simulink model "simulation_model"  (R2019b)
settings: Solver=VariableStepAuto  StartTime=0.0  StopTime=3  RelTol=1e-3
values from neighbouring files (symbols this model uses):
  g = 9.80665    [main.m]
  h = 0.5    [main.m]
  kv = 0.1    [main.m]
  m = 30 * 10^-3    (= 0.03)    [main.m]
  v0_x = v0 * cos(theta)    [main.m]
  v0_y = v0 * sin(theta)    [main.m]
libraries: simulink x1
settings Model: Creator=super  LastModifiedBy=super

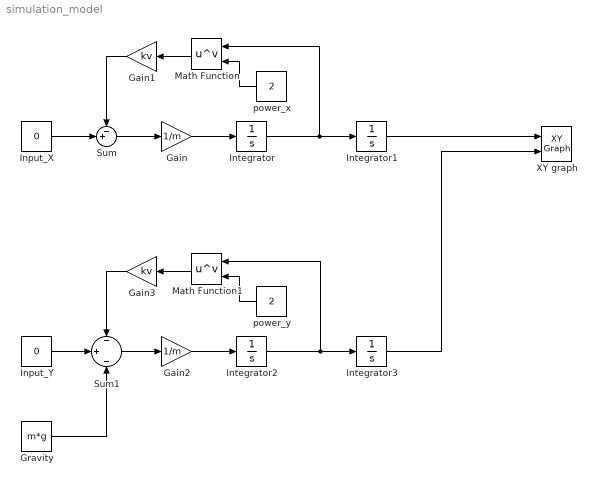
== system simulation_model ==
  Gain : Gain  Gain=1/m
  Gain1 : Gain  Gain=kv
  Gain2 : Gain  Gain=1/m
  Gain3 : Gain  Gain=kv
  Gravity : Constant  Value=m*g
  Input_X : Constant  Value=0
  Input_Y : Constant  Value=0
  Integrator : Integrator  InitialCondition=v0_x  LimitOutput=on  LowerSaturationLimit=0
  Integrator1 : Integrator
  Integrator2 : Integrator  InitialCondition=v0_y  LimitOutput=on  UpperSaturationLimit=10^3  LowerSaturationLimit=-10^3
  Integrator3 : Integrator  InitialCondition=h  LimitOutput=on  LowerSaturationLimit=0
  Math Function : Math  Operator=pow  SignedPower=off  SaturateOnIntegerOverflow=on
  Math Function1 : Math  Operator=pow  SignedPower=off  SaturateOnIntegerOverflow=on
  Sum : Sum  Inputs=-+|
  Sum1 : Sum  Inputs=-|+|-
  XY graph : simulink/Sinks/XY Graph  xmin=-1  xmax=5  ymin=0  ymax=1  st=-1
  power_x : Constant  Value=2
  power_y : Constant  Value=2
  wires:
  Sum/1 -> Gain/1
  Input_X/1 -> Sum/2
  Gain/1 -> Integrator/1
  Integrator/1 -> Math Function/1, Integrator1/1
  power_x/1 -> Math Function/2
  Math Function/1 -> Gain1/1
  Gain1/1 -> Sum/1
  Math Function1/1 -> Gain3/1
  power_y/1 -> Math Function1/2
  Gain2/1 -> Integrator2/1
  Integrator2/1 -> Math Function1/1, Integrator3/1
  Sum1/1 -> Gain2/1
  Gain3/1 -> Sum1/1
  Integrator3/1 -> XY graph/2
  Input_Y/1 -> Sum1/2
  Gravity/1 -> Sum1/3
  Integrator1/1 -> XY graph/1
